simulink model "LED_BBB_Driver"  (R2015a)
settings: Solver=ode15s  StartTime=0.0  StopTime=5  RelTol=1e-5
libraries: fl_lib x20, nesl_utility x9, elec_lib x1
settings Model: Creator=peer23peer  LastModifiedBy=peer23peer
settings SimscapeCC: SimscapeLogType=all  SimscapeLogSimulationStatistics=on  SimscapeLogOpenViewer=on

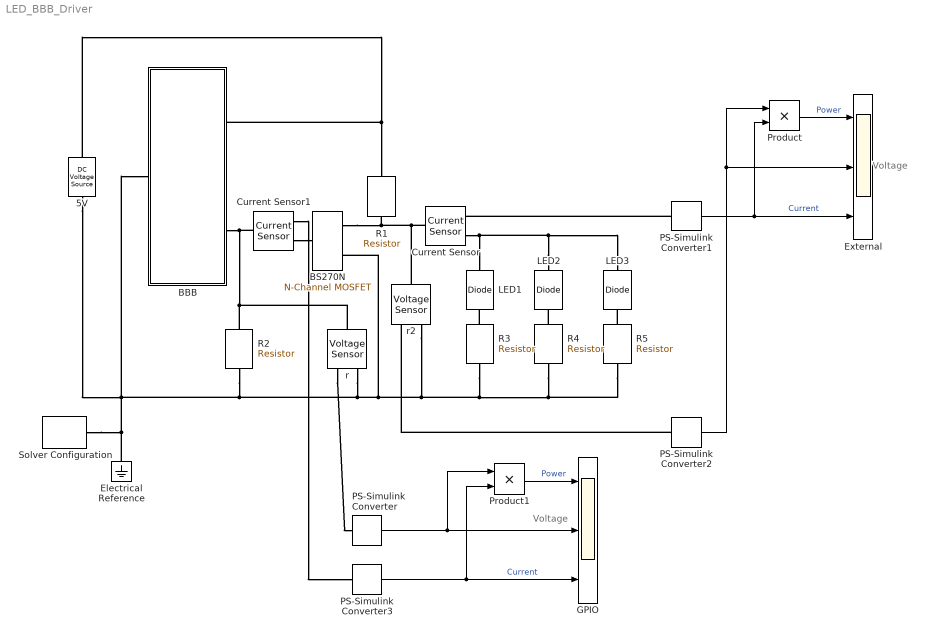
== system LED_BBB_Driver ==
  note: Voltage
  note: Voltage
  5V : fl_lib/Electrical/Electrical Sources/DC Voltage Source  v0=5 V
  BBB : Subsystem
  BS270N : elec_lib/Semiconductor Devices/N-Channel MOSFET  parameterization=1  prmDatasheet=2  prmEquCoeff=1  Beta=5 A/V^2  Rds=3.5 Ohm  Id=600 mA  Vgs=4.5 V  Vth=2.5 V  lam=0 1/V  Tmeas=25 C  RS=1e-4 Ohm  RD=0.01 Ohm  C_param=1  C_GS=270 pF  C_GD=80 pF  C_iss=50 pF  C_rss=5 pF  C_oss=25 pF  C_GS_vec=[ 270 300 290 280 295 255 ] pF  C_GD_vec=[ 450 400 300 190 95 55 ] pF  C_iss_vec=[ 720 700 590 470 390 310 ] pF  C_rss_vec=[ 450 400 300 190 95 55 ] pF  C_oss_vec=[ 900 810 690 420 270 170 ] pF  C_Vds_vec=[ 0.1 0.3 1 3 10 30 ] V  charge_linearity_param=1  C_OX=200 pF  V_C_OX=-0.5 V  dVth_dT=-6 mV/K  Rds_T2=3.5 Ohm  Tmeas2=125 C  BEXDatasheet=-1.5  BEXEquCoeff=-1.5  TdeviceDatasheet=25 C  TdeviceEquCoeff=25 C  Rth=[ 0 10 ] K/W  thermal_mass_parameterization=1  thermal_mass=[ 0 1 ] J/K  thermal_time_constant=[ 0 10 ] s  thermal_mass_initial_temperatures=[ 25 25 ] C
      settings: LogSimulationData=on
  Current Sensor : fl_lib/Electrical/Electrical Sensors/Current Sensor
  Current Sensor1 : fl_lib/Electrical/Electrical Sensors/Current Sensor
  Electrical Reference : fl_lib/Electrical/Electrical Elements/Electrical Reference
  External : Scope  NumInputPorts=3
      settings: ShowLegends=on  YMin=5.55112e-17~0~1.38778e-17  YMax=0.9~4~0.25  SaveName=ScopeData2
  GPIO : Scope  NumInputPorts=3
      settings: ShowLegends=on  YMin=-25~0~-25  YMax=150~3.5~175
  LED1 : fl_lib/Electrical/Electrical Elements/Diode  Vf=3.4 V  Ron=0.3 Ohm  Goff=1e-8 1/Ohm  i_specify=on  i_priority=High  i=600 mA  v_specify=off  v_priority=High  v=0 V
      settings: LogSimulationData=on
  LED2 : fl_lib/Electrical/Electrical Elements/Diode  Vf=3.4 V  Ron=0.3 Ohm  Goff=1e-8 1/Ohm  i_specify=on  i_priority=High  i=600 mA  v_specify=off  v_priority=High  v=0 V
      settings: LogSimulationData=on
  LED3 : fl_lib/Electrical/Electrical Elements/Diode  Vf=3.4 V  Ron=0.3 Ohm  Goff=1e-8 1/Ohm  i_specify=on  i_priority=High  i=600 mA  v_specify=off  v_priority=High  v=0 V
      settings: LogSimulationData=on
  PS-Simulink Converter : nesl_utility/PS-Simulink Converter  PhysicalDomain=network_engine_domain  SubClassName=ps_output  LeftPortType=input  RightPortType=output  PseudoPeriodic=off  Frequencies=[]  Unit=1  AffineConversion=off
  PS-Simulink Converter1 : nesl_utility/PS-Simulink Converter  PhysicalDomain=network_engine_domain  SubClassName=ps_output  LeftPortType=input  RightPortType=output  PseudoPeriodic=off  Frequencies=[]  Unit=1  AffineConversion=off
  PS-Simulink Converter2 : nesl_utility/PS-Simulink Converter  PhysicalDomain=network_engine_domain  SubClassName=ps_output  LeftPortType=input  RightPortType=output  PseudoPeriodic=off  Frequencies=[]  Unit=V  AffineConversion=off
  PS-Simulink Converter3 : nesl_utility/PS-Simulink Converter  PhysicalDomain=network_engine_domain  SubClassName=ps_output  LeftPortType=input  RightPortType=output  PseudoPeriodic=off  Frequencies=[]  Unit=1  AffineConversion=off
  Product : Product
  Product1 : Product
  R1 : fl_lib/Electrical/Electrical Elements/Resistor  R=100 Ohm  i_specify=off  i_priority=High  i=0 A  v_specify=off  v_priority=High  v=0 V
  R2 : fl_lib/Electrical/Electrical Elements/Resistor  R=1 MOhm  i_specify=off  i_priority=High  i=0 A  v_specify=off  v_priority=High  v=0 V
  R3 : fl_lib/Electrical/Electrical Elements/Resistor  R=7 Ohm  i_specify=off  i_priority=High  i=0 A  v_specify=off  v_priority=High  v=0 V
  R4 : fl_lib/Electrical/Electrical Elements/Resistor  R=7 Ohm  i_specify=off  i_priority=High  i=0 A  v_specify=off  v_priority=High  v=0 V
  R5 : fl_lib/Electrical/Electrical Elements/Resistor  R=7 Ohm  i_specify=off  i_priority=High  i=0 A  v_specify=off  v_priority=High  v=0 V
  Solver Configuration : nesl_utility/Solver Configuration  PhysicalDomain=network_engine_domain  SubClassName=solver  LeftPortType=input  RightPortType=generic  Accelerate=off  Tones=[]  Harmonics=[]  SimulateNoise=off  Profile=off  UseLocalSampling=off  EnableSwitchedLinearOptims=on  FrequencyDomain=off  UseCCode=off  RelTol=0.001  AbsTol=1e-06  MinStep=1e-09  ToWorkspace=off  RevertToSquareIcSolve=off  NumHomotopyIterations=100  DoDC=off  ResidualTolerance=1e-09  UseLocalSolver=off  LocalSolverChoice=NE_BACKWARD_EULER_ADVANCER  LocalSolverSampleTime=0.001  DoFixedCost=off  MaxNonlinIter=3  MaxModeIter=2  LinearAlgebra=Sparse  DelaysMemoryBudget=1024  AutomaticFiltering=on  FilteringTimeConstant=0.001
  r : fl_lib/Electrical/Electrical Sensors/Voltage Sensor
  r2 : fl_lib/Electrical/Electrical Sensors/Voltage Sensor
  wires:
  PS-Simulink Converter1/1 -> Product/2, External/3  "Current"
  PS-Simulink Converter2/1 -> External/2, Product/1
  Product/1 -> External/1  "Power"
  PS-Simulink Converter3/1 -> Product1/2, GPIO/3  "Current"
  PS-Simulink Converter/1 -> Product1/1, GPIO/2
  Product1/1 -> GPIO/1  "Power"
  connections:
  BS270N/RConn2 -- r2/RConn2 -- R5/RConn1 -- R4/RConn1 -- R3/RConn1 -- R2/LConn1 -- Solver Configuration/RConn1 -- Electrical Reference/LConn1 -- BBB/LConn1 -- 5V/RConn1 -- r/RConn2
  BBB/RConn2 -- r/LConn1 -- R2/RConn1 -- Current Sensor1/LConn1
  PS-Simulink Converter2/LConn1 -- r2/RConn1
  LED2/LConn1 -- LED3/LConn1 -- Current Sensor/RConn2 -- LED1/LConn1
  R4/LConn1 -- LED2/RConn1
  R5/LConn1 -- LED3/RConn1
  R3/LConn1 -- LED1/RConn1
  5V/LConn1 -- R1/RConn1 -- BBB/RConn1
  r/RConn1 -- PS-Simulink Converter/LConn1
  r2/LConn1 -- Current Sensor/LConn1 -- BS270N/RConn1 -- R1/LConn1
  Current Sensor1/RConn2 -- BS270N/LConn1
  PS-Simulink Converter1/LConn1 -- Current Sensor/RConn1
  Current Sensor1/RConn1 -- PS-Simulink Converter3/LConn1

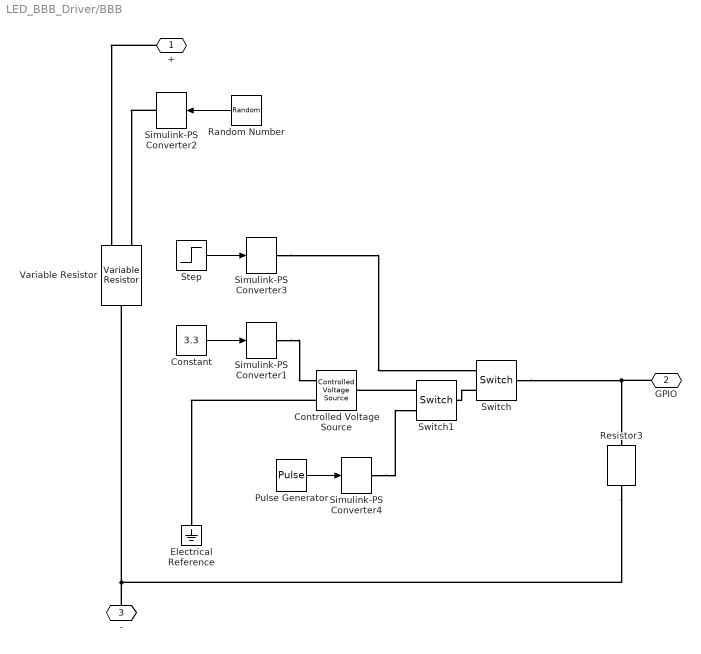
== system LED_BBB_Driver/BBB ==
  Constant : Constant  Value=3.3
  Controlled Voltage Source : fl_lib/Electrical/Electrical Sources/Controlled Voltage Source
  Electrical Reference : fl_lib/Electrical/Electrical Elements/Electrical Reference
  Pulse Generator : DiscretePulseGenerator  PulseType=Time based  Period=1/100  PulseWidth=99
  Random Number : RandomNumber  Mean=13  Variance=3  Seed=534  SampleTime=0.2
  Resistor3 : fl_lib/Electrical/Electrical Elements/Resistor  R=20 kOhm  i_specify=off  i_priority=High  i=0 A  v_specify=off  v_priority=High  v=0 V
  Simulink-PS Converter{1..4} (4 alike) : nesl_utility/Simulink-PS Converter  PhysicalDomain=network_engine_domain  SubClassName=ps_input  LeftPortType=input  RightPortType=output  PseudoPeriodic=off  Frequencies=[]  NoiseDistribution=none  NoiseParameters=[]  Unit=1  AffineConversion=off  InputFiltering=off  SimscapeFilterOrder=1  InputFilterTimeConstant=0.001  UdotUserProvided=1
  Step : Step  Time=3  SampleTime=0
  Switch : fl_lib/Electrical/Electrical Elements/Switch  R_closed=0.01 Ohm  G_open=1e-8 1/Ohm  Threshold=0  i_specify=off  i_priority=High  i=0 A  v_specify=off  v_priority=High  v=0 V
  Switch1 : fl_lib/Electrical/Electrical Elements/Switch  R_closed=0.01 Ohm  G_open=1e-8 1/Ohm  Threshold=0  i_specify=off  i_priority=High  i=0 A  v_specify=off  v_priority=High  v=0 V
  Variable Resistor : fl_lib/Electrical/Electrical Elements/Variable Resistor  Rmin=0 Ohm  i_specify=off  i_priority=High  i=0 A  v_specify=off  v_priority=High  v=0 V
  + : PMIOPort  Port=1  Side=Right
  GPIO : PMIOPort  Port=2  Side=Right
  - : PMIOPort  Port=3  Side=Left
  wires:
  Random Number/1 -> Simulink-PS Converter2/1
  Constant/1 -> Simulink-PS Converter1/1
  Step/1 -> Simulink-PS Converter3/1
  Pulse Generator/1 -> Simulink-PS Converter4/1
  connections:
  Simulink-PS Converter2/RConn1 -- Variable Resistor/LConn1
  +/RConn1 -- Variable Resistor/LConn2
  -/RConn1 -- Variable Resistor/RConn1 -- Resistor3/RConn1
  Simulink-PS Converter1/RConn1 -- Controlled Voltage Source/RConn1
  Controlled Voltage Source/RConn2 -- Electrical Reference/LConn1
  Simulink-PS Converter3/RConn1 -- Switch/RConn1
  Switch1/RConn2 -- Controlled Voltage Source/LConn1
  Switch/RConn2 -- Switch1/LConn1
  Switch/LConn1 -- GPIO/RConn1 -- Resistor3/LConn1
  Simulink-PS Converter4/RConn1 -- Switch1/RConn1
